simulink model "Death_star"  (R2025a)
settings: Solver=VariableStepAuto  StartTime=0.0  StopTime=50  RelTol=1e-3
model workspace: external: MAT-File C:\Users\alexa1\Desktop\cox\tueind\bep_stuff\simulation\with_added_3Dprints\Simscape\Death_star_DataFile.mat (data not in the file)
values from neighbouring files (symbols this model uses):
  air_bearing = struct    [Death_star_DataFile.m]
  camera = struct    [Death_star_DataFile.m]
  deathstar = struct    [Death_star_DataFile.m]
  gravity = 0    [Death_star_DataFile.m]
  Init_cond_motor_angular_rate_rpm = 50/Kff * 60/(2*pi)    (= 6689.28225815)    [Death_star_DataFile.m]
  J_motor = (smiData.Solid(1).MoI(2) + smiData.Solid(2).MoI(2))*(1e-6)    [Death_star_DataFile.m]
  kd_pitch = k_deg * 0.01    (= 1.14591559026)    [Death_star_DataFile.m]
  kd_yaw = k_deg * 0.02    (= 2.29183118052)    [Death_star_DataFile.m]
  Kff = 1/14.01    (= 0.0713775874375)    [Death_star_DataFile.m]    (also in inner_loop_test.m = 0.0714285714286)
  ki_pitch = k_deg * 0.01    (= 1.14591559026)    [Death_star_DataFile.m]
  ki_yaw = k_deg * 0.01    (= 1.14591559026)    [Death_star_DataFile.m]
  Kp = 0    [Death_star_DataFile.m]    (also in inner_loop_test.m)
  kp_pitch = k_deg * 5    (= 572.957795131)    [Death_star_DataFile.m]
  kp_yaw = k_deg * 5    (= 572.957795131)    [Death_star_DataFile.m]
  laser = struct    [Death_star_DataFile.m]
  N = length(time)    [torqueThrottle.m]
  noise = 0    [Death_star_DataFile.m]
  smiData = struct    [Death_star_DataFile.m]
  tf_den = sys_tf.Denominator    [Death_star_DataFile.m]
  tf_num = sys_tf.Numerator    [Death_star_DataFile.m]
  throttle_offset = 0    [Death_star_DataFile.m]    (also in torqueThrottle.m = 50)
  Ts = sys_tf.Ts    [Death_star_DataFile.m]    (also in inner_loop_test.m = 0.02; torqueThrottle.m = 0.02)
undefined symbols (not defined in the file or in its folder): DiscIntNeverNeededParam, dspblkCoreblockFVToolHelper, gcbh, Init_cond_motor_angular_rate, X, Y, Z
libraries: sm_lib x39, nesl_utility x29, slpidlib x7, simulink x5, aerolibutil x4, matrix_library x3, sharedutil x2
(part 1 of 2)
settings Model: SimulationMode=accelerator  Creator=20211194  LastModifiedBy=alexa1
settings ExplorerConfigSet: InternalSimMechanicsExplorerSettings=|
  | <ExplorerConfiguration>
  | 
  |   <canonicalview>default</canonicalview>
  | 
  |   <TilePanel>
  |     <TileInfo>
  |       <Tiles Columns="1" Count="1" Height="984" Rows="1" Width="1142">
  |         <Row Weight="1"/>
  |         <Column Weight="1"/>
  |         <Tile Height="1" Width="1" X="0" Y="0"/>
  |       </Tiles>
  |     </TileInfo>
  |     <SceneInfo>
  |       <SceneViewer>
  |         <IsThisViewStd>
  |           <IsStandardView>off</IsStandardView>
  |           <StandardViewName>Front</StandardViewName>
  |         </IsThisViewStd>
  |         <BGColor>
  |           <R>1</R>
  |           <G>1</G>
  |           <B>1</B>
  |           <A>1</A>
  |         </BGColor>
  |         <Camera>
  |           <DoPerspective>off</DoPerspective>
  |           <Position>
  |             <X>6.226265641035277</X>
  |             <Y>0</Y>
  |             <Z>-0.0081156130875740112</Z>
  |           </Position>
  |           <Center>
  |             <X>0.73991890804263705</X>
  |             <Y>0</Y>
  |             <Z>-0.0081156130875740112</Z>
  |           </Center>
  |           <Up>
  |             <X>0</X>
  |             <Y>0</Y>
  |             <Z>1</Z>
  |           </Up>
  |           <XLim>0.18753742752712968</XLim>
  |           <YLim>0.071004529966450514</YLim>
  |           <ViewLimDist>0.01</ViewLimDist>
  |         </Camera>
  |       </SceneViewer>
  |     </SceneInfo>
  |   </TilePanel>
  | 
  |   <MechEditorPanel>
  |     <GfxPanelCameraMap/>
  |     <Cameras/>
  |     <VideoCreator>
  |       <IncludeTiles>All</IncludeTiles>
  |       <IncludeTime>on</IncludeTime>
  |       <IncludeWorldFrame>off</IncludeWorldFrame>
  |       <PlaybackSpeedRatio>1</PlaybackSpeedRatio>
  |       <FrameRate>30</FrameRate>
  |       <FrameSize>auto</FrameSize>
  |       <VideoFormat>MotionJPEGAVI</VideoFormat>
  |     </VideoCreator>
  |   </MechEditorPanel>
  | 
  |   <PlaybackSettings>
  |     <PlaybackSpeedFactor>32</PlaybackSpeedFactor>
  |   </PlaybackSettings>
  | 
  | </ExplorerConfiguration>

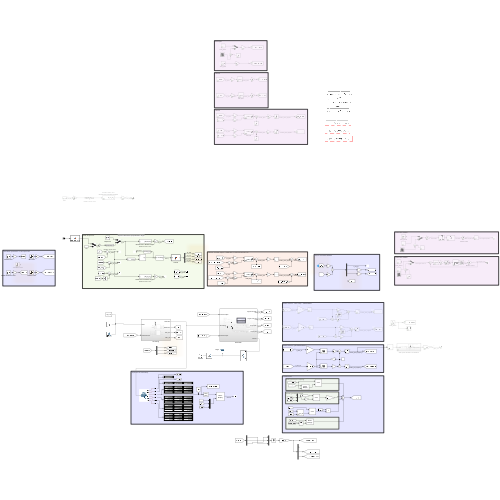
[thumbnail: Simulink's stored preview of the top-level diagram]
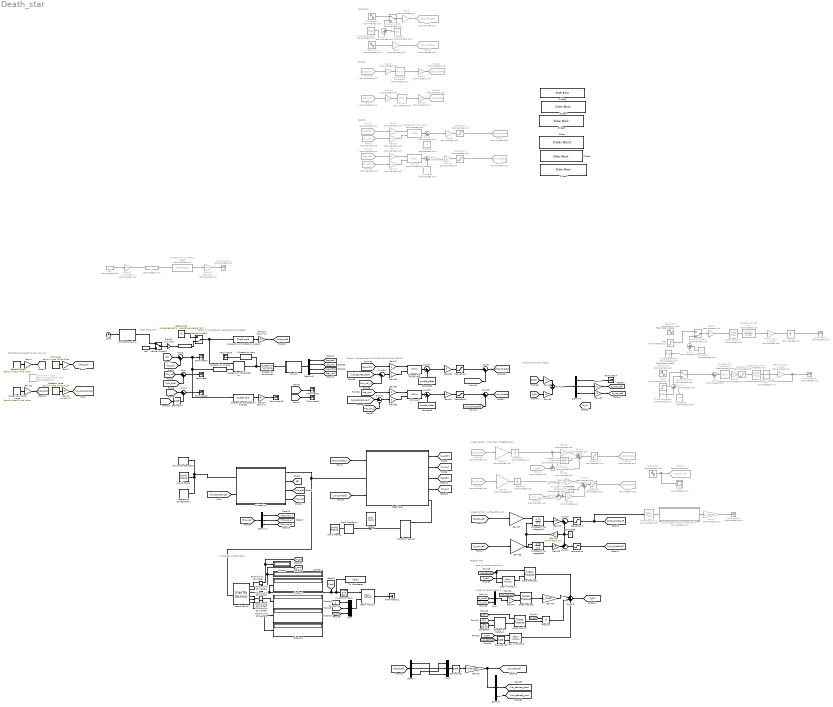
== system Death_star ==
  note: torque command wheels
  note: properties of total setup
  note: wheel gyroscopic torque
  note: body gyroscopic coupling
  note: Feedforward
  note: Wheel control - inner loop + feedforward
  note: setpoint is laser-beam perpendicular to target
  note: Data acquisition
  note: Stochastic processes: to be improved
  note: Control
  note: Test input
  note: Test motor model
  note: Control
  note: Test motor model
  note: Wheel control - just feedforward
  note: Control - throttle output - SIMILAR TO PHYSICAL SETUP
  " " : Angle2Quat
      settings: AttributesFormatString=Rotation Order: %<rotationOrder>
  " 1" : Angle2Quat  Commented=on
      settings: AttributesFormatString=Rotation Order: %<rotationOrder>
  Air bearing : Subsystem
      settings: PortSchema="{\"entries\":[{\"content\":{\"sides\":[{\"content\":{\"connectorIds\":[\"LConn1\",\"In1\"]},\"type\":\"ConnectorPlacement.EquallySpacedRectSide\",\"uuid\":\"0635cb36-f09f-446f-95ef-83ab4fad6854\"},{\"content\":{\"connectorIds\":[\"RConn1\",\"Out1\",\"Out2\",\"Out3\"],\"side\":\"RIGHT\"},\"type\":\"ConnectorPlacement.EquallySpacedRectSide\",\"uuid\":\"d78ff47b-39b0-4ee7-b059-0862b1f53b89\"},{\"content\":{\"side\":\"TOP\"},\"type\":\"ConnectorPlacement.EquallySpacedRectSide\",\"uuid\":\"7d14a825-fa15-4e78-b928-77825eb00abd\"}]},\"type\":\"ConnectorPlacement.EquallySpacedConnector\",\"uuid\":\"d18951ee-81c9-4a51-8692-d921bd8b40bf\"}],\"packageUris\":[\"http://schema.mathworks.com/mf0/Connector/R2020b\"],\"version\":\"1.0\"}"
  Camera noise : simulink/Sources/Band-Limited White Noise  Cov=camera_noise  Ts=0.1  seed=[777]
  Clock : Clock
  Constant : Constant  Commented=on  Value=30
  Constant1 : Constant  Commented=on  Value=-15
  Constant2 : Constant  Commented=on  Value=0
  Constant3 : Constant  Commented=on  Value=0
  Constant4 : Constant  Value=0
  Constant5 : Constant  Commented=on  Value=-15
  Constant6 : Constant  Value=0
  Constant7 : Constant  Value=[0 0 -gravity]
  Constant8 : Constant  Value=throttle_offset
  Constant9 : Constant  Value=throttle_offset
  Cross Product : matrix_library/Cross Product
  Cross Product1 : matrix_library/Cross Product
  Cross Product2 : matrix_library/Cross Product
  Death Star : Subsystem
      settings: PortSchema="{\"entries\":[{\"content\":{\"sides\":[{\"content\":{\"connectorIds\":[\"In1\",\"LConn1\",\"In2\"]},\"type\":\"ConnectorPlacement.EquallySpacedRectSide\",\"uuid\":\"6976bf24-5cda-40d9-bbe9-3c1c1e8447ae\"},{\"content\":{\"connectorIds\":[\"Out1\",\"Out2\",\"Out3\",\"Out4\",\"RConn1\"],\"side\":\"RIGHT\"},\"type\":\"ConnectorPlacement.EquallySpacedRectSide\",\"uuid\":\"d5b6db99-c631-425f-aa61-45b10154e4c7\"},{\"content\":{\"side\":\"TOP\"},\"type\":\"ConnectorPlacement.EquallySpacedRectSide\",\"uuid\":\"3ba9b0f3-1c65-4336-998e-243dd9c30860\"}]},\"type\":\"ConnectorPlacement.EquallySpacedConnector\",\"uuid\":\"830a7446-c9c8-4228-9816-4bf4fdd904e1\"}],\"packageUris\":[\"http://schema.mathworks.com/mf0/Connector/R2020b\"],\"version\":\"1.0\"}"
  Demux{,1..2,4} (4 alike) : Demux  Outputs=3
  Demux3 : Demux
  Derivative : Derivative
  Derivative1 : Derivative
  Derivative2 : Derivative
  Discrete Transfer Fcn : DiscreteTransferFcn  Commented=on  LoadFcn=dspblkCoreblockFVToolHelper(gcbh,'load');  Numerator=tf_num  Denominator=tf_den
      settings: CopyFcn=dspblkCoreblockFVToolHelper(gcbh,'copy');  DeleteFcn=dspblkCoreblockFVToolHelper(gcbh,'close');  ModelCloseFcn=dspblkCoreblockFVToolHelper(gcbh,'close');  PreSaveFcn=dspblkCoreblockFVToolHelper(gcbh,'presave');  PostSaveFcn=dspblkCoreblockFVToolHelper(gcbh,'postsave');  CloseFcn=dspblkCoreblockFVToolHelper(gcbh,'close');
  Discrete Transfer Fcn1 : DiscreteTransferFcn  Commented=on  LoadFcn=dspblkCoreblockFVToolHelper(gcbh,'load');  Numerator=tf_num  Denominator=tf_den
      settings: CopyFcn=dspblkCoreblockFVToolHelper(gcbh,'copy');  DeleteFcn=dspblkCoreblockFVToolHelper(gcbh,'close');  ModelCloseFcn=dspblkCoreblockFVToolHelper(gcbh,'close');  PreSaveFcn=dspblkCoreblockFVToolHelper(gcbh,'presave');  PostSaveFcn=dspblkCoreblockFVToolHelper(gcbh,'postsave');  CloseFcn=dspblkCoreblockFVToolHelper(gcbh,'close');
  Discrete PID Controller : slpidlib/PID Controller  Commented=on  Controller=PID  Form=Parallel  TimeDomain=Discrete-time  UseExternalTs=off  SampleTime=0.02  IntegratorMethod=Forward Euler  FilterMethod=Forward Euler  ControllerParametersSource=internal  P=kp_pitch  I=ki_pitch  UseKiTs=off  D=kd_pitch  UseExternalDerivativeSource=on  N=20  UseFilter=on  TunerSelectOption=Transfer Function Based (PID Tuner App)  InitialConditionSource=internal  InitialConditionForIntegrator=0  InitialConditionForFilter=0  DifferentiatorICPrevScaledInput=0  ExternalReset=none  TrackingMode=off  Kt=1  LimitOutput=on  SatLimitsSource=internal  UpperSaturationLimit=25  LowerSaturationLimit=-25  LinearizeAsGain=off  AntiWindupMode=clamping  Kb=1  LimitIntegrator=off  UpperIntegratorSaturationLimit=inf  LowerIntegratorSaturationLimit=-inf  POutMin=[]  POutMax=[]  IOutMin=[]  IOutMax=[]  DOutMin=[]  DOutMax=[]  NOutMin=[]  NOutMax=[]  SumOutMin=[]  SumOutMax=[]  SaturationOutMin=[]  SaturationOutMax=[]  PParamMin=[]  PParamMax=[]  IParamMin=[]  IParamMax=[]  DParamMin=[]  DParamMax=[]  NParamMin=[]  NParamMax=[]  KbParamMin=[]  KbParamMax=[]  KtParamMin=[]  KtParamMax=[]  KbOutMin=[]  KbOutMax=[]  KtOutMin=[]  KtOutMax=[]  IntegratorOutMin=[]  IntegratorOutMax=[]  FilterOutMin=[]  FilterOutMax=[]  SumI1OutMin=[]  SumI1OutMax=[]  SumI2OutMin=[]  SumI2OutMax=[]  SumI3OutMin=[]  SumI3OutMax=[]  SumI4OutMin=[]  SumI4OutMax=[]  SumDOutMin=[]  SumDOutMax=[]  DifferentiatorOutMin=[]  DifferentiatorOutMax=[]  FilterDiffOutCoefMin=[]  FilterDiffOutCoefMax=[]  ReciprocalOutMin=[]  ReciprocalOutMax=[]  SumDenOutMin=[]  SumDenOutMax=[]  SumNumOutMin=[]  SumNumOutMax=[]  DivideOutMin=[]  DivideOutMax=[]  UdiffTsProdOutMin=[]  UdiffTsProdOutMax=[]  NTsProdOutMin=[]  NTsProdOutMax=[]  UintegralTsProdOutMin=[]  UintegralTsProdOutMax=[]  UngainTsProdOutMin=[]  UngainTsProdOutMax=[]  ClampingZeroOutDataTypeStr=Inherit: Inherit via back propagation  ClampingZeroOutMin=[]  ClampingZeroOutMax=[]  FilterDenConstantOutDataTypeStr=Inherit: Inherit via back propagation  FilterDenConstantOutMin=[]  FilterDenConstantOutMax=[]  PCopyOutDataTypeStr=Inherit: Inherit via back propagation  PCopyOutMin=[]  PCopyOutMax=[]  NCopyOutDataTypeStr=Inherit: Inherit via back propagation  NCopyOutMin=[]  NCopyOutMax=[]  IntegratorContinuousStateAttributes=''  IntegratorStateMustResolveToSignalObject=off  IntegratorRTWStateStorageClass=Auto  FilterContinuousStateAttributes=''  FilterStateMustResolveToSignalObject=off  FilterRTWStateStorageClass=Auto  ParallelPVariant=InternalParameters  IdealPVariant=Disabled  IVariant=InternalParameters  DVariant=InternalParameters  IntegratorVariant=Discrete  SatVariant=Enabled  AWVariant=DiscClampingParallel  PCopyVariant=Disabled  TRVariant=Disabled  FdbkBlocksVariant=Forward  IdealPFdbkVariant=Disabled  SatFdbkVariant=Disabled  DerivativeFilterVariant=ForwardEulerFilterOnly  NVariant=InternalParameters  NCopyVariant=Disabled  FilterICVariant=InternalICsFilter  IntegratorICVariant=InternalICs  ExternalResetVariant=Disabled  TRSumVariant=Passthrough  SumFdbkVariant=Disabled  SumVariant=Sum_PID  TsampFilterVariant=InternalTs  TsampNgainVariant=Passthrough  TsampIntegralVariant=Disabled_SignalSpec  ExternalSaturationOutDataTypeStr=Inherit: Same as second input  DerivativeSourceVariant=ExternalYdot  PreIntVariant=InternalPreInt
      settings: LibrarySourceBlock=simulink/Discrete/Discrete PID Controller
  Discrete PID Controller1 : slpidlib/PID Controller  Commented=on  Controller=PID  Form=Parallel  TimeDomain=Discrete-time  UseExternalTs=off  SampleTime=0.02  IntegratorMethod=Forward Euler  FilterMethod=Forward Euler  ControllerParametersSource=internal  P=kp_pitch  I=ki_pitch  UseKiTs=off  D=kd_pitch  UseExternalDerivativeSource=off  N=20  UseFilter=on  TunerSelectOption=Transfer Function Based (PID Tuner App)  InitialConditionSource=internal  InitialConditionForIntegrator=0  InitialConditionForFilter=0  DifferentiatorICPrevScaledInput=0  ExternalReset=none  TrackingMode=off  Kt=1  LimitOutput=off  SatLimitsSource=internal  UpperSaturationLimit=inf  LowerSaturationLimit=-inf  LinearizeAsGain=off  AntiWindupMode=none  Kb=1  LimitIntegrator=off  UpperIntegratorSaturationLimit=inf  LowerIntegratorSaturationLimit=-inf  POutMin=[]  POutMax=[]  IOutMin=[]  IOutMax=[]  DOutMin=[]  DOutMax=[]  NOutMin=[]  NOutMax=[]  SumOutMin=[]  SumOutMax=[]  SaturationOutMin=[]  SaturationOutMax=[]  PParamMin=[]  PParamMax=[]  IParamMin=[]  IParamMax=[]  DParamMin=[]  DParamMax=[]  NParamMin=[]  NParamMax=[]  KbParamMin=[]  KbParamMax=[]  KtParamMin=[]  KtParamMax=[]  KbOutMin=[]  KbOutMax=[]  KtOutMin=[]  KtOutMax=[]  IntegratorOutMin=[]  IntegratorOutMax=[]  FilterOutMin=[]  FilterOutMax=[]  SumI1OutMin=[]  SumI1OutMax=[]  SumI2OutMin=[]  SumI2OutMax=[]  SumI3OutMin=[]  SumI3OutMax=[]  SumI4OutMin=[]  SumI4OutMax=[]  SumDOutMin=[]  SumDOutMax=[]  DifferentiatorOutMin=[]  DifferentiatorOutMax=[]  FilterDiffOutCoefMin=[]  FilterDiffOutCoefMax=[]  ReciprocalOutMin=[]  ReciprocalOutMax=[]  SumDenOutMin=[]  SumDenOutMax=[]  SumNumOutMin=[]  SumNumOutMax=[]  DivideOutMin=[]  DivideOutMax=[]  UdiffTsProdOutMin=[]  UdiffTsProdOutMax=[]  NTsProdOutMin=[]  NTsProdOutMax=[]  UintegralTsProdOutMin=[]  UintegralTsProdOutMax=[]  UngainTsProdOutMin=[]  UngainTsProdOutMax=[]  ClampingZeroOutDataTypeStr=Inherit: Inherit via back propagation  ClampingZeroOutMin=[]  ClampingZeroOutMax=[]  FilterDenConstantOutDataTypeStr=Inherit: Inherit via back propagation  FilterDenConstantOutMin=[]  FilterDenConstantOutMax=[]  PCopyOutDataTypeStr=Inherit: Inherit via back propagation  PCopyOutMin=[]  PCopyOutMax=[]  NCopyOutDataTypeStr=Inherit: Inherit via back propagation  NCopyOutMin=[]  NCopyOutMax=[]  IntegratorContinuousStateAttributes=''  IntegratorStateMustResolveToSignalObject=off  IntegratorRTWStateStorageClass=Auto  FilterContinuousStateAttributes=''  FilterStateMustResolveToSignalObject=off  FilterRTWStateStorageClass=Auto  ParallelPVariant=InternalParameters  IdealPVariant=Disabled  IVariant=InternalParameters  DVariant=InternalParameters  IntegratorVariant=Discrete  SatVariant=Disabled  AWVariant=Passthrough  PCopyVariant=Disabled  TRVariant=Disabled  FdbkBlocksVariant=Forward  IdealPFdbkVariant=Disabled  SatFdbkVariant=Disabled  DerivativeFilterVariant=ForwardEulerFilter  NVariant=InternalParameters  NCopyVariant=Disabled  FilterICVariant=InternalICsFilter  IntegratorICVariant=InternalICs  ExternalResetVariant=Disabled  TRSumVariant=Passthrough  SumFdbkVariant=Disabled  SumVariant=Sum_PID  TsampFilterVariant=InternalTs  TsampNgainVariant=Passthrough  TsampIntegralVariant=Disabled_SignalSpec  ExternalSaturationOutDataTypeStr=Inherit: Same as second input  DerivativeSourceVariant=ErrorSignal  PreIntVariant=InternalPreInt
      settings: LibrarySourceBlock=simulink/Discrete/Discrete PID Controller
  Discrete PID Controller2 : slpidlib/PID Controller  Commented=on  Controller=PID  Form=Parallel  TimeDomain=Discrete-time  UseExternalTs=off  SampleTime=-1  IntegratorMethod=Forward Euler  FilterMethod=Forward Euler  ControllerParametersSource=internal  P=1  I=0  UseKiTs=off  D=0  UseExternalDerivativeSource=off  N=100  UseFilter=on  TunerSelectOption=Transfer Function Based (PID Tuner App)  InitialConditionSource=internal  InitialConditionForIntegrator=0  InitialConditionForFilter=0  DifferentiatorICPrevScaledInput=0  ExternalReset=none  TrackingMode=off  Kt=1  LimitOutput=off  SatLimitsSource=internal  UpperSaturationLimit=inf  LowerSaturationLimit=-inf  LinearizeAsGain=off  AntiWindupMode=none  Kb=1  LimitIntegrator=off  UpperIntegratorSaturationLimit=inf  LowerIntegratorSaturationLimit=-inf  POutMin=[]  POutMax=[]  IOutMin=[]  IOutMax=[]  DOutMin=[]  DOutMax=[]  NOutMin=[]  NOutMax=[]  SumOutMin=[]  SumOutMax=[]  SaturationOutMin=[]  SaturationOutMax=[]  PParamMin=[]  PParamMax=[]  IParamMin=[]  IParamMax=[]  DParamMin=[]  DParamMax=[]  NParamMin=[]  NParamMax=[]  KbParamMin=[]  KbParamMax=[]  KtParamMin=[]  KtParamMax=[]  KbOutMin=[]  KbOutMax=[]  KtOutMin=[]  KtOutMax=[]  IntegratorOutMin=[]  IntegratorOutMax=[]  FilterOutMin=[]  FilterOutMax=[]  SumI1OutMin=[]  SumI1OutMax=[]  SumI2OutMin=[]  SumI2OutMax=[]  SumI3OutMin=[]  SumI3OutMax=[]  SumI4OutMin=[]  SumI4OutMax=[]  SumDOutMin=[]  SumDOutMax=[]  DifferentiatorOutMin=[]  DifferentiatorOutMax=[]  FilterDiffOutCoefMin=[]  FilterDiffOutCoefMax=[]  ReciprocalOutMin=[]  ReciprocalOutMax=[]  SumDenOutMin=[]  SumDenOutMax=[]  SumNumOutMin=[]  SumNumOutMax=[]  DivideOutMin=[]  DivideOutMax=[]  UdiffTsProdOutMin=[]  UdiffTsProdOutMax=[]  NTsProdOutMin=[]  NTsProdOutMax=[]  UintegralTsProdOutMin=[]  UintegralTsProdOutMax=[]  UngainTsProdOutMin=[]  UngainTsProdOutMax=[]  ClampingZeroOutDataTypeStr=Inherit: Inherit via back propagation  ClampingZeroOutMin=[]  ClampingZeroOutMax=[]  FilterDenConstantOutDataTypeStr=Inherit: Inherit via back propagation  FilterDenConstantOutMin=[]  FilterDenConstantOutMax=[]  PCopyOutDataTypeStr=Inherit: Inherit via back propagation  PCopyOutMin=[]  PCopyOutMax=[]  NCopyOutDataTypeStr=Inherit: Inherit via back propagation  NCopyOutMin=[]  NCopyOutMax=[]  IntegratorContinuousStateAttributes=''  IntegratorStateMustResolveToSignalObject=off  IntegratorRTWStateStorageClass=Auto  FilterContinuousStateAttributes=''  FilterStateMustResolveToSignalObject=off  FilterRTWStateStorageClass=Auto  ParallelPVariant=InternalParameters  IdealPVariant=Disabled  IVariant=InternalParameters  DVariant=InternalParameters  IntegratorVariant=Discrete  SatVariant=Disabled  AWVariant=Passthrough  PCopyVariant=Disabled  TRVariant=Disabled  FdbkBlocksVariant=Forward  IdealPFdbkVariant=Disabled  SatFdbkVariant=Disabled  DerivativeFilterVariant=ForwardEulerFilter  NVariant=InternalParameters  NCopyVariant=Disabled  FilterICVariant=InternalICsFilter  IntegratorICVariant=InternalICs  ExternalResetVariant=Disabled  TRSumVariant=Passthrough  SumFdbkVariant=Disabled  SumVariant=Sum_PID  TsampFilterVariant=InternalTs  TsampNgainVariant=Passthrough  TsampIntegralVariant=Disabled_SignalSpec  ExternalSaturationOutDataTypeStr=Inherit: Same as second input  DerivativeSourceVariant=ErrorSignal  PreIntVariant=InternalPreInt
      settings: LibrarySourceBlock=simulink/Discrete/Discrete PID Controller
  Discrete PID Controller3 : slpidlib/PID Controller  Controller=PID  Form=Parallel  TimeDomain=Discrete-time  UseExternalTs=off  SampleTime=0.02  IntegratorMethod=Forward Euler  FilterMethod=Forward Euler  ControllerParametersSource=internal  P=kp_pitch  I=ki_pitch  UseKiTs=on  D=kd_pitch  UseExternalDerivativeSource=on  N=20  UseFilter=on  TunerSelectOption=Transfer Function Based (PID Tuner App)  InitialConditionSource=internal  InitialConditionForIntegrator=0  InitialConditionForFilter=0  DifferentiatorICPrevScaledInput=0  ExternalReset=none  TrackingMode=off  Kt=1  LimitOutput=on  SatLimitsSource=internal  UpperSaturationLimit=25  LowerSaturationLimit=-25  LinearizeAsGain=off  AntiWindupMode=clamping  Kb=1  LimitIntegrator=off  UpperIntegratorSaturationLimit=inf  LowerIntegratorSaturationLimit=-inf  POutMin=[]  POutMax=[]  IOutMin=[]  IOutMax=[]  DOutMin=[]  DOutMax=[]  NOutMin=[]  NOutMax=[]  SumOutMin=[]  SumOutMax=[]  SaturationOutMin=[]  SaturationOutMax=[]  PParamMin=[]  PParamMax=[]  IParamMin=[]  IParamMax=[]  DParamMin=[]  DParamMax=[]  NParamMin=[]  NParamMax=[]  KbParamMin=[]  KbParamMax=[]  KtParamMin=[]  KtParamMax=[]  KbOutMin=[]  KbOutMax=[]  KtOutMin=[]  KtOutMax=[]  IntegratorOutMin=[]  IntegratorOutMax=[]  FilterOutMin=[]  FilterOutMax=[]  SumI1OutMin=[]  SumI1OutMax=[]  SumI2OutMin=[]  SumI2OutMax=[]  SumI3OutMin=[]  SumI3OutMax=[]  SumI4OutMin=[]  SumI4OutMax=[]  SumDOutMin=[]  SumDOutMax=[]  DifferentiatorOutMin=[]  DifferentiatorOutMax=[]  FilterDiffOutCoefMin=[]  FilterDiffOutCoefMax=[]  ReciprocalOutMin=[]  ReciprocalOutMax=[]  SumDenOutMin=[]  SumDenOutMax=[]  SumNumOutMin=[]  SumNumOutMax=[]  DivideOutMin=[]  DivideOutMax=[]  UdiffTsProdOutMin=[]  UdiffTsProdOutMax=[]  NTsProdOutMin=[]  NTsProdOutMax=[]  UintegralTsProdOutMin=[]  UintegralTsProdOutMax=[]  UngainTsProdOutMin=[]  UngainTsProdOutMax=[]  ClampingZeroOutDataTypeStr=Inherit: Inherit via back propagation  ClampingZeroOutMin=[]  ClampingZeroOutMax=[]  FilterDenConstantOutDataTypeStr=Inherit: Inherit via back propagation  FilterDenConstantOutMin=[]  FilterDenConstantOutMax=[]  PCopyOutDataTypeStr=Inherit: Inherit via back propagation  PCopyOutMin=[]  PCopyOutMax=[]  NCopyOutDataTypeStr=Inherit: Inherit via back propagation  NCopyOutMin=[]  NCopyOutMax=[]  IntegratorContinuousStateAttributes=''  IntegratorStateMustResolveToSignalObject=off  IntegratorRTWStateStorageClass=Auto  FilterContinuousStateAttributes=''  FilterStateMustResolveToSignalObject=off  FilterRTWStateStorageClass=Auto  ParallelPVariant=InternalParameters  IdealPVariant=Disabled  IVariant=InternalParameters  DVariant=InternalParameters  IntegratorVariant=Discrete  SatVariant=Enabled  AWVariant=DiscClampingParallel  PCopyVariant=Disabled  TRVariant=Disabled  FdbkBlocksVariant=Forward  IdealPFdbkVariant=Disabled  SatFdbkVariant=Disabled  DerivativeFilterVariant=ForwardEulerFilterOnly  NVariant=InternalParameters  NCopyVariant=Disabled  FilterICVariant=InternalICsFilter  IntegratorICVariant=InternalICs  ExternalResetVariant=Disabled  TRSumVariant=Passthrough  SumFdbkVariant=Disabled  SumVariant=Sum_PID  TsampFilterVariant=InternalTs  TsampNgainVariant=Passthrough  TsampIntegralVariant=Disabled_SignalSpec  ExternalSaturationOutDataTypeStr=Inherit: Same as second input  DerivativeSourceVariant=ExternalYdot  PreIntVariant=InternalPreInt
      settings: LibrarySourceBlock=simulink/Discrete/Discrete PID Controller
  Discrete-Time Integrator : DiscreteIntegrator  Commented=on  gainval=Ki  SampleTime=-1  ICPrevOutput=DiscIntNeverNeededParam  ICPrevScaledInput=DiscIntNeverNeededParam
  Discrete-Time Integrator1 : DiscreteIntegrator  Commented=on  gainval=Ki  SampleTime=-1  ICPrevOutput=DiscIntNeverNeededParam  ICPrevScaledInput=DiscIntNeverNeededParam
  Discrete-Time Integrator2 : DiscreteIntegrator  InitialConditionSource=external  InitialCondition=Init_cond_motor_angular_rate_rpm  SampleTime=Ts  ICPrevOutput=DiscIntNeverNeededParam  ICPrevScaledInput=DiscIntNeverNeededParam
  Discrete-Time Integrator3 : DiscreteIntegrator  InitialConditionSource=external  InitialCondition=Init_cond_motor_angular_rate_rpm  SampleTime=Ts  ICPrevOutput=DiscIntNeverNeededParam  ICPrevScaledInput=DiscIntNeverNeededParam
  Display{,1..5} (6 alike) : Display
  From11 : From  Commented=on  GotoTag=qe_pitch
  From12 : From  Commented=on  GotoTag=qe_yaw
  From13 : From  Commented=on  GotoTag=qe_pitch
  From14 : From  Commented=on  GotoTag=qe_yaw
  From16 : From  Commented=on  GotoTag=IMU_vel_z
  From17 : From  Commented=on  GotoTag=IMU_vel_y
  From24 : From  Commented=on  GotoTag=w_pitch
  From25 : From  Commented=on  GotoTag=w_yaw
  From28 : From  Commented=on  GotoTag=t_pitch_ref
  From29 : From  Commented=on  GotoTag=t_yaw_ref
  Gain{,1,3,5,9..11,19} (8 alike) : Gain  Commented=on
  Gain{12..13,20..21} (4 alike) : Gain  Commented=on  Gain=-1
  Gain14 : Gain  Gain=360/(2*pi)
  Gain15 : Gain  Gain=360/(2*pi)
  Gain16 : Gain  Commented=on  Gain=360/(2*pi)
  Gain17 : Gain  Commented=on  Gain=(2*pi)/360
  Gain18 : Gain  Gain=(2*pi)/360
  Gain2 : Gain  Commented=on  Gain=0
  Gain22 : Gain  Gain=noise
  Gain23 : Gain  Gain=(2*pi)/360
  Gain27 : Gain  Commented=on  Gain=J_motor
  Gain29 : Gain  Commented=on  Gain=Kff
  Gain30 : Gain  Commented=on  Gain=Kp
  Gain31 : Gain  Commented=on  Gain=Kff
  Gain32 : Gain  Commented=on  Gain=Kp
  Gain33 : Gain  Gain=Kff
  Gain34 : Gain  Commented=on  Gain=1/J_motor
  Gain35 : Gain  Gain=Kff
  Gain36 : Gain  Commented=on  Gain=1/J_motor
  Gain37 : Gain  Gain=1/J_motor
  Gain38 : Gain  Gain=1/J_motor
  Gain4 : Gain  Gain=noise
  Gain40 : Gain  Gain=(1/Kff)*(60/(2*pi))
  Gain43 : Gain  Gain=J_motor
  Gain{44,46..48} (4 alike) : Gain  Gain=-1
  Gain{45,56..61} (7 alike) : Gain
  Gain6 : Gain  Gain=noise*0+1
  Gain7 : Gain  Gain=noise
  Gain8 : Gain  Commented=on  Gain=0
  Goto{8,10,15,26} (4 alike) : Goto  Commented=on  GotoTag=yaw_throttle
  Goto{7,9,14,25} (4 alike) : Goto  Commented=on  GotoTag=pitch_throttle
  Goto27 : Goto  Commented=on  GotoTag=t_pitch_ref
  IMU noise : simulink/Sources/Band-Limited White Noise  Cov=imu_noise  Ts=0.01  seed=[77]
  Inertia Sensor : sm_lib/Body Elements/Inertia Sensor  SensorExtent=Mechanism  SpanWeldJoints=on  ExcludeGroundedBodies=off  MeasurementFrame=Attached  SenseMass=on  SenseCenterOfMass=on  SenseInertiaMatrix=on  SenseCenteredInertiaMatrix=on  SensePrincipalInertiaMatrix=on  SenseRotationMatrix=on  GraphicType=PrincipalInertiaFrame  PrincipalInertiaFrameSize=20  GraphicVisPropType=SimpleVisualProperties  GraphicDiffuseColor=[0.5 0.5 0.5]  GraphicOpacity=1  GraphicSpecularColor=[0.5 0.5 0.5 1.0]  GraphicAmbientColor=[0.15 0.15 0.15 1.0]  GraphicEmissiveColor=[0.0 0.0 0.0 1.0]  GraphicShininess=75
  Integrator : Integrator  Commented=on
  Integrator1 : Integrator  Commented=on  InitialCondition=Init_cond_motor_angular_rate
  Integrator2 : Integrator  Commented=on  InitialCondition=Init_cond_motor_angular_rate
  Invert 3x3 Matrix : aerolibutil/Invert  3x3 Matrix
  MATLAB Function1 : MATLAB Function  TreatAsAtomicUnit=on
  Manual Switch : ManualSwitch  Commented=on
  Manual Switch1 : ManualSwitch  Commented=on  CurrentSetting=0
  Manual Switch2 : ManualSwitch  CurrentSetting=0
  Manual Switch3 : ManualSwitch  Commented=on
  Manual Switch4 : ManualSwitch
  Matrix Multiply : Product  Multiplication=Matrix(*)
  Matrix Multiply1 : Product  Multiplication=Matrix(*)
  Matrix Multiply2 : Product  Multiplication=Matrix(*)
  Mechanism Configuration : sm_lib/Utilities/Mechanism Configuration  UniformGravity=Constant  GravityVector=[0 0 -gravity]  GravityVectorUnits=m/s^2  LinearizationDelta=0.001  JointModeTransitionNonlinearIterations=2
  Mux : Mux  Inputs=3
  Mux1 : Mux  Inputs=3
  Mux2 : Mux  Inputs=3
  PID yaw : slpidlib/PID Controller  Commented=on  Controller=PID  Form=Parallel  TimeDomain=Discrete-time  UseExternalTs=off  SampleTime=0.02  IntegratorMethod=Forward Euler  FilterMethod=Forward Euler  ControllerParametersSource=internal  P=454.5454545454545  I=0  UseKiTs=off  D=2.1127  UseExternalDerivativeSource=on  N=20  UseFilter=on  TunerSelectOption=Transfer Function Based (PID Tuner App)  InitialConditionSource=internal  InitialConditionForIntegrator=0  InitialConditionForFilter=0  DifferentiatorICPrevScaledInput=0  ExternalReset=none  TrackingMode=off  Kt=1  LimitOutput=on  SatLimitsSource=internal  UpperSaturationLimit=25  LowerSaturationLimit=-25  LinearizeAsGain=off  AntiWindupMode=clamping  Kb=1  LimitIntegrator=off  UpperIntegratorSaturationLimit=inf  LowerIntegratorSaturationLimit=-inf  POutMin=[]  POutMax=[]  IOutMin=[]  IOutMax=[]  DOutMin=[]  DOutMax=[]  NOutMin=[]  NOutMax=[]  SumOutMin=[]  SumOutMax=[]  SaturationOutMin=[]  SaturationOutMax=[]  PParamMin=[]  PParamMax=[]  IParamMin=[]  IParamMax=[]  DParamMin=[]  DParamMax=[]  NParamMin=[]  NParamMax=[]  KbParamMin=[]  KbParamMax=[]  KtParamMin=[]  KtParamMax=[]  KbOutMin=[]  KbOutMax=[]  KtOutMin=[]  KtOutMax=[]  IntegratorOutMin=[]  IntegratorOutMax=[]  FilterOutMin=[]  FilterOutMax=[]  SumI1OutMin=[]  SumI1OutMax=[]  SumI2OutMin=[]  SumI2OutMax=[]  SumI3OutMin=[]  SumI3OutMax=[]  SumI4OutMin=[]  SumI4OutMax=[]  SumDOutMin=[]  SumDOutMax=[]  DifferentiatorOutMin=[]  DifferentiatorOutMax=[]  FilterDiffOutCoefMin=[]  FilterDiffOutCoefMax=[]  ReciprocalOutMin=[]  ReciprocalOutMax=[]  SumDenOutMin=[]  SumDenOutMax=[]  SumNumOutMin=[]  SumNumOutMax=[]  DivideOutMin=[]  DivideOutMax=[]  UdiffTsProdOutMin=[]  UdiffTsProdOutMax=[]  NTsProdOutMin=[]  NTsProdOutMax=[]  UintegralTsProdOutMin=[]  UintegralTsProdOutMax=[]  UngainTsProdOutMin=[]  UngainTsProdOutMax=[]  ClampingZeroOutDataTypeStr=Inherit: Inherit via back propagation  ClampingZeroOutMin=[]  ClampingZeroOutMax=[]  FilterDenConstantOutDataTypeStr=Inherit: Inherit via back propagation  FilterDenConstantOutMin=[]  FilterDenConstantOutMax=[]  PCopyOutDataTypeStr=Inherit: Inherit via back propagation  PCopyOutMin=[]  PCopyOutMax=[]  NCopyOutDataTypeStr=Inherit: Inherit via back propagation  NCopyOutMin=[]  NCopyOutMax=[]  IntegratorContinuousStateAttributes=''  IntegratorStateMustResolveToSignalObject=off  IntegratorRTWStateStorageClass=Auto  FilterContinuousStateAttributes=''  FilterStateMustResolveToSignalObject=off  FilterRTWStateStorageClass=Auto  ParallelPVariant=InternalParameters  IdealPVariant=Disabled  IVariant=InternalParameters  DVariant=InternalParameters  IntegratorVariant=Discrete  SatVariant=Enabled  AWVariant=DiscClampingParallel  PCopyVariant=Disabled  TRVariant=Disabled  FdbkBlocksVariant=Forward  IdealPFdbkVariant=Disabled  SatFdbkVariant=Disabled  DerivativeFilterVariant=ForwardEulerFilterOnly  NVariant=InternalParameters  NCopyVariant=Disabled  FilterICVariant=InternalICsFilter  IntegratorICVariant=InternalICs  ExternalResetVariant=Disabled  TRSumVariant=Passthrough  SumFdbkVariant=Disabled  SumVariant=Sum_PID  TsampFilterVariant=InternalTs  TsampNgainVariant=Passthrough  TsampIntegralVariant=Disabled_SignalSpec  ExternalSaturationOutDataTypeStr=Inherit: Same as second input  DerivativeSourceVariant=ExternalYdot  PreIntVariant=InternalPreInt
      settings: LibrarySourceBlock=simulink/Discrete/Discrete PID Controller
  PID yaw1 : slpidlib/PID Controller  Commented=on  Controller=PID  Form=Parallel  TimeDomain=Discrete-time  UseExternalTs=off  SampleTime=0.02  IntegratorMethod=Forward Euler  FilterMethod=Forward Euler  ControllerParametersSource=internal  P=703.1733746130031  I=0  UseKiTs=off  D=0  UseExternalDerivativeSource=off  N=20  UseFilter=on  TunerSelectOption=Transfer Function Based (PID Tuner App)  InitialConditionSource=internal  InitialConditionForIntegrator=0  InitialConditionForFilter=0  DifferentiatorICPrevScaledInput=0  ExternalReset=none  TrackingMode=off  Kt=1  LimitOutput=off  SatLimitsSource=internal  UpperSaturationLimit=inf  LowerSaturationLimit=-inf  LinearizeAsGain=off  AntiWindupMode=none  Kb=1  LimitIntegrator=off  UpperIntegratorSaturationLimit=inf  LowerIntegratorSaturationLimit=-inf  POutMin=[]  POutMax=[]  IOutMin=[]  IOutMax=[]  DOutMin=[]  DOutMax=[]  NOutMin=[]  NOutMax=[]  SumOutMin=[]  SumOutMax=[]  SaturationOutMin=[]  SaturationOutMax=[]  PParamMin=[]  PParamMax=[]  IParamMin=[]  IParamMax=[]  DParamMin=[]  DParamMax=[]  NParamMin=[]  NParamMax=[]  KbParamMin=[]  KbParamMax=[]  KtParamMin=[]  KtParamMax=[]  KbOutMin=[]  KbOutMax=[]  KtOutMin=[]  KtOutMax=[]  IntegratorOutMin=[]  IntegratorOutMax=[]  FilterOutMin=[]  FilterOutMax=[]  SumI1OutMin=[]  SumI1OutMax=[]  SumI2OutMin=[]  SumI2OutMax=[]  SumI3OutMin=[]  SumI3OutMax=[]  SumI4OutMin=[]  SumI4OutMax=[]  SumDOutMin=[]  SumDOutMax=[]  DifferentiatorOutMin=[]  DifferentiatorOutMax=[]  FilterDiffOutCoefMin=[]  FilterDiffOutCoefMax=[]  ReciprocalOutMin=[]  ReciprocalOutMax=[]  SumDenOutMin=[]  SumDenOutMax=[]  SumNumOutMin=[]  SumNumOutMax=[]  DivideOutMin=[]  DivideOutMax=[]  UdiffTsProdOutMin=[]  UdiffTsProdOutMax=[]  NTsProdOutMin=[]  NTsProdOutMax=[]  UintegralTsProdOutMin=[]  UintegralTsProdOutMax=[]  UngainTsProdOutMin=[]  UngainTsProdOutMax=[]  ClampingZeroOutDataTypeStr=Inherit: Inherit via back propagation  ClampingZeroOutMin=[]  ClampingZeroOutMax=[]  FilterDenConstantOutDataTypeStr=Inherit: Inherit via back propagation  FilterDenConstantOutMin=[]  FilterDenConstantOutMax=[]  PCopyOutDataTypeStr=Inherit: Inherit via back propagation  PCopyOutMin=[]  PCopyOutMax=[]  NCopyOutDataTypeStr=Inherit: Inherit via back propagation  NCopyOutMin=[]  NCopyOutMax=[]  IntegratorContinuousStateAttributes=''  IntegratorStateMustResolveToSignalObject=off  IntegratorRTWStateStorageClass=Auto  FilterContinuousStateAttributes=''  FilterStateMustResolveToSignalObject=off  FilterRTWStateStorageClass=Auto  ParallelPVariant=InternalParameters  IdealPVariant=Disabled  IVariant=InternalParameters  DVariant=InternalParameters  IntegratorVariant=Discrete  SatVariant=Disabled  AWVariant=Passthrough  PCopyVariant=Disabled  TRVariant=Disabled  FdbkBlocksVariant=Forward  IdealPFdbkVariant=Disabled  SatFdbkVariant=Disabled  DerivativeFilterVariant=ForwardEulerFilter  NVariant=InternalParameters  NCopyVariant=Disabled  FilterICVariant=InternalICsFilter  IntegratorICVariant=InternalICs  ExternalResetVariant=Disabled  TRSumVariant=Passthrough  SumFdbkVariant=Disabled  SumVariant=Sum_PID  TsampFilterVariant=InternalTs  TsampNgainVariant=Passthrough  TsampIntegralVariant=Disabled_SignalSpec  ExternalSaturationOutDataTypeStr=Inherit: Same as second input  DerivativeSourceVariant=ErrorSignal  PreIntVariant=InternalPreInt
      settings: LibrarySourceBlock=simulink/Discrete/Discrete PID Controller
  PID yaw2 : slpidlib/PID Controller  Controller=PID  Form=Parallel  TimeDomain=Discrete-time  UseExternalTs=off  SampleTime=0.02  IntegratorMethod=Forward Euler  FilterMethod=Forward Euler  ControllerParametersSource=internal  P=kp_yaw  I=ki_yaw  UseKiTs=on  D=kd_yaw  UseExternalDerivativeSource=on  N=20  UseFilter=on  TunerSelectOption=Transfer Function Based (PID Tuner App)  InitialConditionSource=internal  InitialConditionForIntegrator=0  InitialConditionForFilter=0  DifferentiatorICPrevScaledInput=0  ExternalReset=none  TrackingMode=off  Kt=1  LimitOutput=on  SatLimitsSource=internal  UpperSaturationLimit=25  LowerSaturationLimit=-25  LinearizeAsGain=off  AntiWindupMode=clamping  Kb=1  LimitIntegrator=off  UpperIntegratorSaturationLimit=inf  LowerIntegratorSaturationLimit=-inf  POutMin=[]  POutMax=[]  IOutMin=[]  IOutMax=[]  DOutMin=[]  DOutMax=[]  NOutMin=[]  NOutMax=[]  SumOutMin=[]  SumOutMax=[]  SaturationOutMin=[]  SaturationOutMax=[]  PParamMin=[]  PParamMax=[]  IParamMin=[]  IParamMax=[]  DParamMin=[]  DParamMax=[]  NParamMin=[]  NParamMax=[]  KbParamMin=[]  KbParamMax=[]  KtParamMin=[]  KtParamMax=[]  KbOutMin=[]  KbOutMax=[]  KtOutMin=[]  KtOutMax=[]  IntegratorOutMin=[]  IntegratorOutMax=[]  FilterOutMin=[]  FilterOutMax=[]  SumI1OutMin=[]  SumI1OutMax=[]  SumI2OutMin=[]  SumI2OutMax=[]  SumI3OutMin=[]  SumI3OutMax=[]  SumI4OutMin=[]  SumI4OutMax=[]  SumDOutMin=[]  SumDOutMax=[]  DifferentiatorOutMin=[]  DifferentiatorOutMax=[]  FilterDiffOutCoefMin=[]  FilterDiffOutCoefMax=[]  ReciprocalOutMin=[]  ReciprocalOutMax=[]  SumDenOutMin=[]  SumDenOutMax=[]  SumNumOutMin=[]  SumNumOutMax=[]  DivideOutMin=[]  DivideOutMax=[]  UdiffTsProdOutMin=[]  UdiffTsProdOutMax=[]  NTsProdOutMin=[]  NTsProdOutMax=[]  UintegralTsProdOutMin=[]  UintegralTsProdOutMax=[]  UngainTsProdOutMin=[]  UngainTsProdOutMax=[]  ClampingZeroOutDataTypeStr=Inherit: Inherit via back propagation  ClampingZeroOutMin=[]  ClampingZeroOutMax=[]  FilterDenConstantOutDataTypeStr=Inherit: Inherit via back propagation  FilterDenConstantOutMin=[]  FilterDenConstantOutMax=[]  PCopyOutDataTypeStr=Inherit: Inherit via back propagation  PCopyOutMin=[]  PCopyOutMax=[]  NCopyOutDataTypeStr=Inherit: Inherit via back propagation  NCopyOutMin=[]  NCopyOutMax=[]  IntegratorContinuousStateAttributes=''  IntegratorStateMustResolveToSignalObject=off  IntegratorRTWStateStorageClass=Auto  FilterContinuousStateAttributes=''  FilterStateMustResolveToSignalObject=off  FilterRTWStateStorageClass=Auto  ParallelPVariant=InternalParameters  IdealPVariant=Disabled  IVariant=InternalParameters  DVariant=InternalParameters  IntegratorVariant=Discrete  SatVariant=Enabled  AWVariant=DiscClampingParallel  PCopyVariant=Disabled  TRVariant=Disabled  FdbkBlocksVariant=Forward  IdealPFdbkVariant=Disabled  SatFdbkVariant=Disabled  DerivativeFilterVariant=ForwardEulerFilterOnly  NVariant=InternalParameters  NCopyVariant=Disabled  FilterICVariant=InternalICsFilter  IntegratorICVariant=InternalICs  ExternalResetVariant=Disabled  TRSumVariant=Passthrough  SumFdbkVariant=Disabled  SumVariant=Sum_PID  TsampFilterVariant=InternalTs  TsampNgainVariant=Passthrough  TsampIntegralVariant=Disabled_SignalSpec  ExternalSaturationOutDataTypeStr=Inherit: Same as second input  DerivativeSourceVariant=ExternalYdot  PreIntVariant=InternalPreInt
      settings: LibrarySourceBlock=simulink/Discrete/Discrete PID Controller
  PS-Simulink Converter{,1..5} (6 alike) : nesl_utility/PS-Simulink Converter  PhysicalDomain=network_engine_domain  SubClassName=ps_output  LeftPortType=input  RightPortType=output  PseudoPeriodic=off  Frequencies=[]  VectorFormat=inherit  Unit=inherit  AffineConversion=off
  Product : Product
  Pulse Generator : DiscretePulseGenerator  Commented=on  PulseType=Time based  Amplitude=30  Period=4  PulseWidth=50
  Pulse Generator1 : DiscretePulseGenerator  Commented=on  PulseType=Time based  Amplitude=30  Period=0.5  PulseWidth=50
  Pulse Generator2 : DiscretePulseGenerator  Commented=on  PulseType=Time based  Amplitude=30  Period=0.5  PulseWidth=50
  Quaternion Inverse : aerolibutil/Quaternion Inverse
  Quaternion Multiplication : aerolibutil/Quaternion Multiplication
  Quaternion Norm : sharedutil/Quaternion Norm  aMode=aMode
      settings: LibrarySourceBlock=|
      | aerolibutil/Quaternion
      | Norm
  Quaternion Normalize1 : sharedutil/Quaternion Normalize  aMode=aMode
  Quaternion Rotation : aerolibutil/Quaternion Rotation
  Quaternions to Rotation Angles : Quat2Angle
      settings: AttributesFormatString=Rotation Order: %<rotationOrder>
  Quaternions to Rotation Angles1 : Quat2Angle
      settings: AttributesFormatString=Rotation Order: %<rotationOrder>
  Quaternions to Rotation Angles2 : Quat2Angle  Commented=on
      settings: AttributesFormatString=Rotation Order: %<rotationOrder>
  RPM to rad/s : Gain  Commented=on  Gain=2*pi/60
  RPM to rad/s1 : Gain  Commented=on  Gain=2*pi/60
  Rate Transition : RateTransition  Commented=on  OutPortSampleTime=0.02
  Rate Transition1 : RateTransition  Commented=on  OutPortSampleTime=0.02
  Rate Transition2 : RateTransition  Commented=on  OutPortSampleTime=Ts
  Rigid Transform : sm_lib/Frames and Transforms/Rigid Transform  RotationMethod=None  FollAlignAxisA=+X  BaseAlignAxisA=+Y  FollAlignAxisB=+Y  BaseAlignAxisB=+Z  RotationStandardAxis=+Z  RotationAngle=0  RotationAngleUnits=deg  RotationArbitraryAxis=[0 0 1]  RotationSequenceAxes=FollowerAxes  RotationSequence=XYX  RotationSequenceAngles=[0 0 0]  RotationSequenceAnglesUnits=deg  RotationMatrix=[1 0 0;0 1 0;0 0 1]  Quaternion=[1 0 0 0]  TranslationMethod=Cylindrical  TranslationCartesianOffset=[0 0 0]  TranslationCartesianOffsetUnits=m  TranslationStandardAxis=+Z  TranslationStandardOffset=0  TranslationStandardOffsetUnits=m  TranslationROffset=1  TranslationROffsetUnits=m  TranslationThetaOffset=0  TranslationThetaOffsetUnits=deg  TranslationZOffset=0  TranslationZOffsetUnits=cm
  Rotation noise : simulink/Sources/Band-Limited White Noise  Cov=rotation_noise  Ts=0.01  seed=[7]
  Saturation{,1..2,5..6} (5 alike) : Saturate  Commented=on  UpperLimit=100  LowerLimit=-100
  Saturation{3..4,7..8} (4 alike) : Saturate  UpperLimit=100  LowerLimit=-100
  Scope : Scope  Commented=on
      settings: ActiveDisplayYMinimum=-1  ActiveDisplayYMaximum=1
  Slider : SliderBlock  ScaleMax=1000
  Slider1 : SliderBlock
  Slider2 : SliderBlock  ScaleMax=10
  Slider3 : SliderBlock  ScaleMax=1000
  Slider4 : SliderBlock
  Slider5 : SliderBlock  ScaleMax=10
  Solver Configuration : nesl_utility/Solver Configuration  PhysicalDomain=network_engine_domain  SubClassName=solver  LeftPortType=input  RightPortType=generic  Tones=[]  Harmonics=[]  SimulateNoise=off  Profile=off  UseLocalSampling=off  EnableSwitchedLinearOptims=on  FrequencyDomain=off  UseCCode=off  RelTol=0.001  AbsTol=0.001  MinStep=1e-09  ToWorkspace=off  RevertToSquareIcSolve=off  NumHomotopyIterations=100  PhasorMode=off  PhasorModeNumHarmonics=1  ConsistencySolver=NEWTON_XTOL_AFTER_FTOL  IndexReductionMethod=DerivativeReplacement  DoDC=off  ResidualTolerance=1e-09  ConsistencyTolSource=GLOBAL  ConsistencyAbsTol=0.001  ConsistencyRelTol=0.001  ConsistencyTolFactor=0.001  UseLocalSolver=off  LocalSolverChoice=NE_BACKWARD_EULER_ADVANCER  ResolveIndetEquations=on  FunctionEvalNumThread=1  LocalSolverSampleTime=0.001  DoFixedCost=off  MaxNonlinIter=3  MaxModeIter=2  ComputeImpulses=off  ImpulseIterations=2  LinearAlgebra=auto  LinearAlgebraNumThread=0  EquationFormulation=NE_TIME_EF  DelaysMemoryBudget=1024  AutomaticFiltering=on  FilteringTimeConstant=0.001  PartitionStorageMethod=AS_NEEDED  PartitionMemoryBudget=1024  PartitionMethod=ROBUST  MultibodyUseLocalSolver=off  MultibodyLocalSolverChoice=ODE1  MultibodyLocalSolverSampleTime=0.001
  Step : Step  Commented=on  After=50  SampleTime=0
  Step1 : Step  Commented=on  After=50  SampleTime=0
  Sum{,1,4,9..10,15,23..24} (8 alike) : Sum  Inputs=|++
  Sum11 : Sum  Commented=on  Inputs=+-|
  Sum12 : Sum  Commented=on  Inputs=|+++
  Sum13 : Sum  Commented=on  Inputs=+-|
  Sum14 : Sum  Commented=on  Inputs=|+++
  Sum16 : Sum  Inputs=++|
  Sum17 : Sum  Inputs=|+-
  Sum18 : Sum  Inputs=++-+
  Sum19 : Sum
  Sum{2..3,5..7} (5 alike) : Sum  Commented=on  Inputs=|++
  Sum20 : Sum  Inputs=|+-
  Sum8 : Sum  Commented=on  Inputs=|+-
  Target : sm_lib/Body Elements/Brick Solid  BrickDimensions=[1 20 20]  BrickDimensionsUnits=cm  ExportEntireGeometry=off  InertiaType=CalculateFromGeometry  BasedOnType=Density  Density=0  DensityUnits=kg/m^3  Mass=1  MassUnits=kg  CenterOfMass=[0 0 0]  CenterOfMassUnits=m  MomentsOfInertia=[1 1 1]  MomentsOfInertiaUnits=kg*m^2  ProductsOfInertia=[0 0 0]  ProductsOfInertiaUnits=kg*m^2  GraphicType=FromGeometry  MarkerShape=Sphere  MarkerSize=10  GraphicVisPropType=SimpleVisualProperties  GraphicDiffuseColor=[0 0.6667 0]  GraphicOpacity=0.6  GraphicSpecularColor=[0.5 0.5 0.5 1.0]  GraphicAmbientColor=[0.15 0.15 0.15 1.0]  GraphicEmissiveColor=[0.0 0.0 0.0 1.0]  GraphicShininess=75  DoExposeReferenceFrame=on  SerializedFrames=<Frames/>
  Terminator{,1..3,5..7,10,12} (9 alike) : Terminator
  Terminator{4,11,13..14} (4 alike) : Terminator  Commented=on
  Test_pitch1 : Sin  Commented=on  Amplitude=20  Frequency=0.1  SampleTime=0
  Test_pitch2 : Sin  Commented=on  Amplitude=20  Frequency=0.1  SampleTime=0
  Test_pitch3 : Sin  Commented=on  Amplitude=20  Frequency=0.1  SampleTime=0
  Test_pitch4 : Sin  Commented=on  Amplitude=0.001  SampleTime=0
  Test_yaw1 : Sin  Commented=on  Amplitude=10  Phase=10  SampleTime=0
  To Workspace : ToWorkspace  VariableName=inertia  SaveFormat=Timeseries  SampleTime=-1
  Transform Sensor : sm_lib/Frames and Transforms/Transform Sensor  MeasurementFrame=World  RotationSequence=XYX  SenseAngle=off  SenseAxis=off  SenseQ=on  SenseR=on  SenseRotationSequence=on  SenseOmegaX=off  SenseOmegaY=off  SenseOmegaZ=off  SenseOmega=off  SenseQDot=off  SenseRDot=off  SenseRotationSequenceDot=off  SenseAlphaX=off  SenseAlphaY=off  SenseAlphaZ=off  SenseAlpha=off  SenseQDDot=off  SenseRDDot=off  SenseX=on  SenseY=on  SenseZ=on  SenseXYZ=off  SenseRad=off  SenseAzim=off  SenseDist=off  SenseInc=off  SenseXDot=off  SenseYDot=off  SenseZDot=off  SenseXYZDot=off  SenseRadDot=off  SenseAzimDot=off  SenseDistDot=off  SenseIncDot=off  SenseXDDot=off  SenseYDDot=off  SenseZDDot=off  SenseXYZDDot=off  SenseRadDDot=off  SenseAzimDDot=off  SenseDistDDot=off  SenseIncDDot=off
  Translation noise : simulink/Sources/Band-Limited White Noise  Commented=on  Cov=0.000001.*ones(3,1)  Ts=0.01  seed=[23341]
  Unwind : MATLAB Function  TreatAsAtomicUnit=on
  Wheel hall sensor noise : simulink/Sources/Band-Limited White Noise  Cov=hall_sens_noise  Ts=0.1  seed=[777]
  World Frame : sm_lib/Frames and Transforms/World Frame
  World Frame1 : sm_lib/Frames and Transforms/World Frame
  set : Constant  Value=[0 -5 0]
  set1 : Constant  Commented=on  Value=[90 0 0]
  setpoint Q1 : Constant  Value=[0.996188036723854, 0.00425790764049721, 0.0871272705745011, 0.000323161005497921]
  state space throttle to acceleration : Subsystem  Commented=on
  wires:
  [Air_disturbance] -> Air bearing/1(Air disturbances)
  Rotation noise/1 -> Gain6/1
  Air bearing/1(Quaternion) -> [Q]
  Air bearing/2(IMU_acc) -> [IMU_acc]
  [IMU_vel] -> Sum/1
  [IMU_dist] -> Sum/2
  Sum/1 -> Terminator/1  "IMU_vel_meas"
  Camera noise/1 -> Gain4/1
  [Q] -> Sum1/1
  [Q_dist] -> Sum1/2
  Sum1/1 -> Quaternion Inverse/1, Quaternions to Rotation Angles1/1, Terminator1/1  "Q_meas"
  Death Star/1(Angular rate pitch) -> [w_pitch]  "omega_m_pitch"
  Death Star/2(Angular rate yaw) -> [w_yaw]  "omega_m_yaw"
  [w_pitch] -> Terminator2/1  "vel_pitch"
  [w_yaw] -> Terminator3/1  "vel_yaw"
  Discrete PID Controller/1 -> Sum6/1
  Gain/1 -> PID yaw/1
  From11/1 -> Gain1/1  "qe_pitch"
  From12/1 -> Gain/1  "qe_yaw"
  [pitch_throttle] -> Death Star/1(Command pitch)
  [yaw_throttle] -> Death Star/2(Command yaw)
  PID yaw/1 -> Sum5/1
  Test_yaw1/1 -> Gain2/1
  Manual Switch/1 -> Gain3/1
  Test_pitch1/1 -> Manual Switch/1
  Constant/1 -> Sum2/2
  Pulse Generator/1 -> Sum2/1
  Sum2/1 -> Manual Switch/2
  Gain3/1 -> Goto9/1
  Discrete Transfer Fcn/1 -> RPM to rad/s/1  "test RPM"
  RPM to rad/s/1 -> Integrator/1  "test angular rate"
  Sum3/1 -> Manual Switch1/2
  Pulse Generator1/1 -> Sum3/1
  Manual Switch1/1 -> Gain5/1
  Gain5/1 -> Rate Transition/1  "test throttle"
  Constant1/1 -> Sum3/2
  Integrator/1 -> Terminator4/1  "test angular position"
  Step/1 -> Manual Switch1/1
  Rate Transition/1 -> Discrete Transfer Fcn/1
  Air bearing/3(IMU_vel) -> [IMU_vel]
  [IMU_acc] -> Sum4/1
  Sum4/1 -> Terminator5/1  "IMU_acc_meas"
  [IMU_dist] -> Derivative/1
  Derivative/1 -> Sum4/2
  Gain4/1 -> [Q_dist]
  Gain6/1 -> [Air_disturbance]
  IMU noise/1 -> Gain7/1
  Gain7/1 -> [IMU_dist]
  Quaternion Multiplication/1 -> Quaternion Normalize1/1, Quaternion Norm/1
  Gain1/1 -> Discrete PID Controller/1
  Gain2/1 -> Goto10/1
  Demux3/4 -> [qe_yaw]  "qe_yaw"
  Demux3/3 -> [qe_pitch]  "qe_pitch"
  Demux3/2 -> [qe_roll]  "qe_roll"
  Quaternion Norm/1 -> Terminator6/1  "norm error"
  Gain8/1 -> Saturation1/1
  Gain9/1 -> Saturation/1
  From13/1 -> Gain11/1  "qe_pitch"
  PID yaw1/1 -> Gain13/1  "throttle_yaw"
  Gain13/1 -> Goto15/1
  Gain12/1 -> Goto14/1
  Gain10/1 -> PID yaw1/1  "position"
  Gain11/1 -> Discrete PID Controller1/1
  From14/1 -> Gain10/1  "qe_yaw"
  Discrete PID Controller1/1 -> Gain12/1  "throttle_pitch"
  Saturation/1 -> Goto8/1  "throttle_yaw_capped"
  Saturation1/1 -> Goto7/1  "throttle_pitch_capped"
  Sum6/1 -> Gain8/1  "throttle_pitch"
  Constant2/1 -> Sum6/2
  Constant3/1 -> Sum5/2
  Sum5/1 -> Gain9/1  "throttle_yaw"
  Manual Switch2/1 -> Quaternion Multiplication/1, Quaternions to Rotation Angles/1  "q_ref"
  Quaternions to Rotation Angles/1 -> Gain15/1
  Demux3/1 -> [qe_scal]  "qe_scal"
  Gain14/1 -> Terminator10/1  "ang_meas"
  Quaternions to Rotation Angles1/1 -> Gain14/1
  Gain15/1 -> [Angle_ref]  "ang_ref"
  setpoint Q1/1 -> Manual Switch2/1
  " "/1 -> Manual Switch2/2
  set1/1 -> Gain17/1  "test_angle_in"
  " 1"/1 -> Quaternions to Rotation Angles2/1
  Quaternions to Rotation Angles2/1 -> Gain16/1
  Gain16/1 -> Terminator11/1  "test_angle_out"
  Gain17/1 -> " 1"/1
  Gain18/1 -> " "/1
  set/1 -> Manual Switch4/2
  [IMU_vel] -> Demux1/1
  Demux1/1 -> [IMU_vel_x]
  Demux1/2 -> [IMU_vel_y]
  Demux1/3 -> [IMU_vel_z]
  From16/1 -> Gain21/1
  From17/1 -> Gain20/1
  PS-Simulink Converter/1 -> [m_tot], Display/1
  PS-Simulink Converter1/1 -> [r_com], Display1/1
  PS-Simulink Converter2/1 -> Display2/1, To Workspace/1, Invert 3x3 Matrix/1, [I_tot]
  PS-Simulink Converter5/1 -> Display5/1
  PS-Simulink Converter3/1 -> Display3/1
  PS-Simulink Converter4/1 -> Display4/1
  Death Star/4(Torque yaw) -> [t_yaw]  "t_yaw"
  Death Star/3(Torque pitch) -> [t_pitch]  "t_pitch"
  Invert 3x3 Matrix/1 -> Matrix Multiply/1
  Mux/1 -> Matrix Multiply/2
  [t_pitch] -> Mux/2
  [t_yaw] -> Mux/3
  Constant4/1 -> Mux/1
  Matrix Multiply/1 -> Terminator12/1  "t_decoup"
  RPM to rad/s1/1 -> Terminator13/1, Sum8/2  "test angular rate"
  Constant5/1 -> Sum7/2
  Step1/1 -> Manual Switch3/1
  Pulse Generator2/1 -> Sum7/1
  Rate Transition1/1 -> Discrete Transfer Fcn1/1
  Discrete Transfer Fcn1/1 -> RPM to rad/s1/1  "test RPM"
  Sum7/1 -> Manual Switch3/2
  Gain19/1 -> Rate Transition1/1  "test throttle"
  Discrete PID Controller2/1 -> Gain19/1
  Manual Switch3/1 -> Sum8/1  "test angular rate ref"
  Sum8/1 -> Discrete PID Controller2/1
  Gain20/1 -> Discrete PID Controller/2
  Gain21/1 -> PID yaw/2
  Wheel hall sensor noise/1 -> Gain22/1
  Gain22/1 -> [hall_dist]
  Saturation5/1 -> Goto25/1  "throttle_pitch_capped"
  Saturation6/1 -> Goto26/1  "throttle_yaw_capped"
  Integrator1/1 -> Sum11/1, Gain29/1
  From24/1 -> Sum11/2
  Sum11/1 -> Discrete-Time Integrator/1, Gain30/1
  Gain30/1 -> Sum12/3
  Gain29/1 -> Sum12/1
  Discrete-Time Integrator/1 -> Sum12/2
  Sum12/1 -> Saturation5/1
  Sum13/1 -> Discrete-Time Integrator1/1, Gain32/1
  Sum14/1 -> Saturation6/1
  Gain31/1 -> Sum14/1
  Discrete-Time Integrator1/1 -> Sum14/2
  Gain32/1 -> Sum14/3
  From25/1 -> Sum13/2
  Saturation7/1 -> Rate Transition2/1, [pitch_throttle_ff]  "throttle_pitch_capped_ff"
  Saturation8/1 -> [yaw_throttle_ff]  "throttle_yaw_capped_ff"
  From28/1 -> Gain34/1  "t_pitch_ref"
  From29/1 -> Gain36/1  "t_yaw_ref"
  Gain34/1 -> Integrator1/1
  Gain36/1 -> Integrator2/1
  Integrator2/1 -> Sum13/1, Gain31/1
  [t_yaw_ref] -> Gain38/1  "t_yaw_ref"
  [t_pitch_ref] -> Gain37/1  "t_pitch_ref"
  Test_pitch4/1 -> Scope/1, Goto27/1
  Gain37/1 -> Discrete-Time Integrator2/1
  state space throttle to acceleration/1(angular accel (rad/s^2)) -> Gain27/1
  Gain27/1 -> Terminator14/1  "t_pitch_out"
  Rate Transition2/1 -> state space throttle to acceleration/1(throttle)
  Gain33/1 -> Sum15/1
  Sum15/1 -> Saturation7/1
  Constant6/1 -> Gain40/1, Sum16/1, Sum15/2
  Gain35/1 -> Sum16/2
  Sum16/1 -> Saturation8/1
  Gain38/1 -> Discrete-Time Integrator3/1
  Discrete-Time Integrator2/1 -> Gain33/1
  Discrete-Time Integrator3/1 -> Gain35/1
  Gain40/1 -> Discrete-Time Integrator2/2, Discrete-Time Integrator3/2
  [vel_desired] -> Matrix Multiply1/2, Cross Product2/1
  [I_tot] -> Matrix Multiply1/1
  Matrix Multiply1/1 -> Cross Product2/2
  Cross Product1/1 -> Gain43/1
  Mux1/1 -> Gain44/1
  Gain44/1 -> Cross Product1/2
  Cross Product2/1 -> Sum18/1
  Gain43/1 -> Sum18/2
  [w_pitch] -> Mux1/2
  [w_yaw] -> Mux1/3
  [Q] -> Quaternion Rotation/1
  Constant7/1 -> Quaternion Rotation/2
  Quaternion Rotation/1 -> Cross Product/2
  [r_com] -> Cross Product/1
  Cross Product/1 -> Product/2
  [m_tot] -> Product/1
  Product/1 -> Sum18/3
  Sum18/1 -> [t_ff]
  Demux4/3 -> Gain48/1
  Demux4/2 -> Gain47/1
  Gain47/1 -> [t_pitch_ref]
  Gain48/1 -> [t_yaw_ref]
  [t_ctrl] -> Gain45/1
  Sum19/1 -> Demux4/1
  [t_ff] -> Gain46/1
  Gain45/1 -> Sum19/1
  Gain46/1 -> Sum19/2
  Demux4/1 -> Terminator7/1  "t_roll_ref"
  Gain60/1 -> Saturation4/1
  Gain59/1 -> PID yaw2/2
  Sum24/1 -> Gain60/1  "throttle_pitch"
  [IMU_vel_z] -> Sum17/2
  PID yaw2/1 -> Sum23/1
  [qe_pitch] -> Gain57/1  "qe_pitch"
  Constant8/1 -> Sum24/2
  Discrete PID Controller3/1 -> Sum24/1
  Saturation3/1 -> Sum10/1  "throttle_yaw_capped"
  [qe_yaw] -> Gain56/1  "qe_yaw"
  Gain61/1 -> Saturation3/1
  Sum23/1 -> Gain61/1  "throttle_yaw"
  Constant9/1 -> Sum23/2
  Saturation4/1 -> Sum9/1  "throttle_pitch_capped"
  Gain57/1 -> Discrete PID Controller3/1
  Gain56/1 -> PID yaw2/1
  [IMU_vel_y] -> Sum20/2
  Gain58/1 -> Discrete PID Controller3/2
  Quaternion Inverse/1 -> Quaternion Multiplication/2
  Quaternion Normalize1/1 -> Unwind/1(qe)  "error q"
  Unwind/1(y) -> Demux3/1
  Clock/1 -> MATLAB Function1/1(t)
  MATLAB Function1/1(y) -> Manual Switch4/1
  Manual Switch4/1 -> Gain18/1  "q_ref"
  Sum9/1 -> [pitch_throttle]  "throttle_pitch"
  [pitch_throttle_ff] -> Sum9/2
  Sum10/1 -> [yaw_throttle]  "throttle_pitch"
  [yaw_throttle_ff] -> Sum10/2
  Gain23/1 -> Demux2/1, [vel_desired]
  Demux/2 -> Mux2/2
  Mux2/1 -> Derivative1/1
  Derivative1/1 -> Gain23/1
  Demux/1 -> Mux2/3
  [Angle_ref] -> Demux/1
  Demux/3 -> Mux2/1
  [vel_desired] -> Cross Product1/1
  [vel_desired] -> Derivative2/1
  Matrix Multiply2/1 -> Sum18/4
  [I_tot] -> Matrix Multiply2/1
  Derivative2/1 -> Matrix Multiply2/2
  Sum17/1 -> Gain59/1  "throttle_pitch"
  Sum20/1 -> Gain58/1  "throttle_pitch"
  Demux2/2 -> [vel_desired_pitch]
  Demux2/3 -> [vel_desired_yaw]
  [vel_desired_pitch] -> Sum20/1
  [vel_desired_yaw] -> Sum17/1
  connections:
  World Frame/RConn1 -- Solver Configuration/RConn1 -- Air bearing/LConn1 -- Mechanism Configuration/RConn1
  Air bearing/RConn1 -- Inertia Sensor/LConn1 -- Death Star/LConn1
  Rigid Transform/LConn1 -- World Frame1/RConn1
  Rigid Transform/RConn1 -- Transform Sensor/LConn1 -- Target/RConn1
  Transform Sensor/RConn1 -- Death Star/RConn1
  PS-Simulink Converter/LConn1 -- Inertia Sensor/RConn1
  PS-Simulink Converter1/LConn1 -- Inertia Sensor/RConn2
  PS-Simulink Converter2/LConn1 -- Inertia Sensor/RConn3
  Inertia Sensor/RConn6 -- PS-Simulink Converter5/LConn1
  Inertia Sensor/RConn5 -- PS-Simulink Converter4/LConn1
  Inertia Sensor/RConn4 -- PS-Simulink Converter3/LConn1
